simulink model "COMPLETO"  (R2024b)
settings: Solver=VariableStepAuto  StartTime=0.0  StopTime=10.0  RelTol=1e-3
undefined symbols (not defined in the file): ih, it, rhd, rtd
settings Model: Creator=ribei  LastModifiedBy=juani

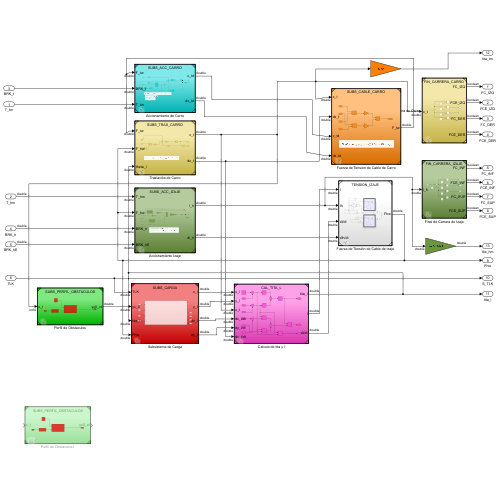
[thumbnail: Simulink's stored preview of the top-level diagram]
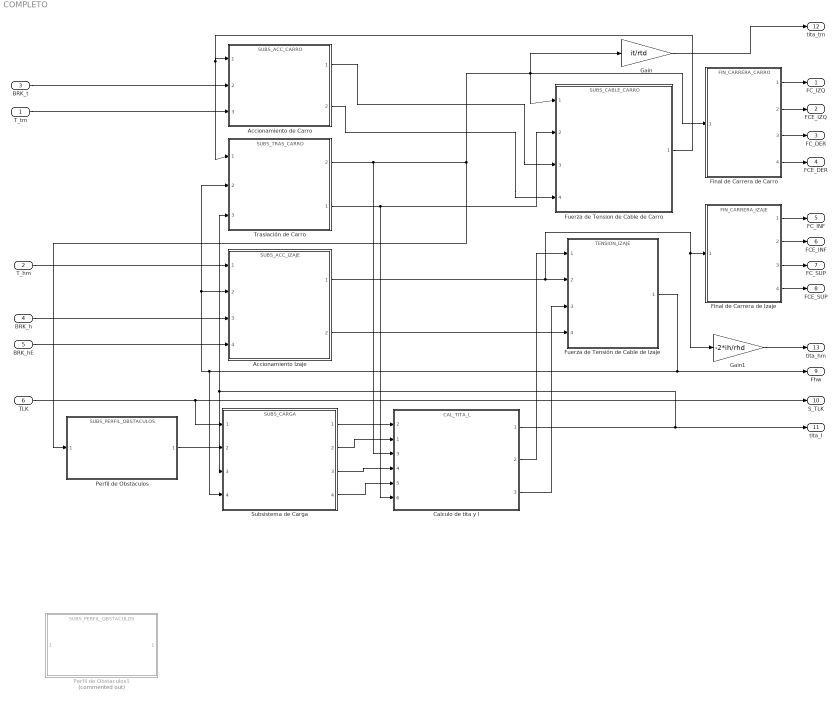
== system COMPLETO ==
  T_tm : Inport
  T_hm : Inport  Port=2
  BRK_t : Inport  Port=3
  BRK_h : Inport  Port=4
  BRK_hE : Inport  Port=5
  TLK : Inport  Port=6
  Accionamiento Izaje : ModelReference  ModelNameDialog=SUBS_ACC_IZAJE.slx  SimulationMode=Normal  ModelReferenceVersion=1.10
  Accionamiento de Carro : ModelReference  ModelNameDialog=SUBS_ACC_CARRO.slx  SimulationMode=Normal  ModelReferenceVersion=1.8
  Calculo de tita y l : ModelReference  ModelNameDialog=CAL_TITA_L.slx  SimulationMode=Normal  ModelReferenceVersion=4.0
      settings: PortSchema="{\"entries\":[{\"content\":{\"sides\":[{\"content\":{\"connectorIds\":[\"In2\",\"In1\",\"In3\",\"In4\",\"In5\",\"In6\"]},\"type\":\"ConnectorPlacement.EquallySpacedRectSide\",\"uuid\":\"8ead184c-a1e0-4b57-8217-57ade3346752\"},{\"content\":{\"connectorIds\":[\"Out1\",\"Out2\",\"Out3\"],\"side\":\"RIGHT\"},\"type\":\"ConnectorPlacement.EquallySpacedRectSide\",\"uuid\":\"562b51b5-55d8-4576-9d04-bf12fcd8d0f5\"},{\"content\":{\"side\":\"TOP\"},\"type\":\"ConnectorPlacement.EquallySpacedRectSide\",\"uuid\":\"2665fda4-9ae8-45ad-8675-5e3ba94dd8e3\"}]},\"type\":\"ConnectorPlacement.EquallySpacedConnector\",\"uuid\":\"240ee59b-efb7-462f-ad93-89fc511299ee\"}],\"packageUris\":[\"http://schema.mathworks.com/mf0/Connector/R2020b\"],\"version\":\"1.0\"}"
  Final de Carrera de Carro : ModelReference  ModelNameDialog=FIN_CARRERA_CARRO.slx  SimulationMode=Normal  ModelReferenceVersion=4.0
  Final de Carrera de Izaje : ModelReference  ModelNameDialog=FIN_CARRERA_IZAJE.slx  SimulationMode=Normal  ModelReferenceVersion=1.1
  Fuerza de Tension de Cable de Carro : ModelReference  ModelNameDialog=SUBS_CABLE_CARRO.slx  SimulationMode=Normal  ModelReferenceVersion=1.2
  Fuerza de Tensión de Cable de Izaje : ModelReference  ModelNameDialog=TENSION_IZAJE.slx  SimulationMode=Normal  ModelReferenceVersion=4.5
  Gain : Gain  Gain=it/rtd
  Gain1 : Gain  Gain=-2*ih/rhd
  Perfil de Obstaculos : ModelReference  ModelNameDialog=SUBS_PERFIL_OBSTACULOS.slx  SimulationMode=Normal  ModelReferenceVersion=1.76
  Perfil de Obstaculos1 : ModelReference  Commented=on  ModelNameDialog=SUBS_PERFIL_OBSTACULOS.slx  SimulationMode=Normal  ModelReferenceVersion=1.75
  Subsistema de Carga : ModelReference  ModelNameDialog=SUBS_CARGA.slx  SimulationMode=Normal  ModelReferenceVersion=1.25
  Traslación de Carro : ModelReference  ModelNameDialog=SUBS_TRAS_CARRO.slx  SimulationMode=Normal  ModelReferenceVersion=1.3
      settings: PortSchema="{\"entries\":[{\"content\":{\"sides\":[{\"content\":{\"connectorIds\":[\"In1\",\"In2\",\"In3\"]},\"type\":\"ConnectorPlacement.EquallySpacedRectSide\",\"uuid\":\"7b046cef-d788-43c7-aa6f-556876391631\"},{\"content\":{\"connectorIds\":[\"Out2\",\"Out1\"],\"side\":\"RIGHT\"},\"type\":\"ConnectorPlacement.EquallySpacedRectSide\",\"uuid\":\"be9a6f00-5e88-4651-bbf2-8ffe22406596\"},{\"content\":{\"side\":\"TOP\"},\"type\":\"ConnectorPlacement.EquallySpacedRectSide\",\"uuid\":\"81b3ad3c-f882-4752-9e65-d53dc15f63b3\"}]},\"type\":\"ConnectorPlacement.EquallySpacedConnector\",\"uuid\":\"5caf2ecc-c1ea-4fc8-a82b-392edb804ace\"}],\"packageUris\":[\"http://schema.mathworks.com/mf0/Connector/R2020b\"],\"version\":\"1.0\"}"
  FC_IZQ : Outport
  FCE_IZQ : Outport  Port=2
  FC_DER : Outport  Port=3
  FCE_DER : Outport  Port=4
  FC_INF : Outport  Port=5
  FCE_INF : Outport  Port=6
  FC_SUP : Outport  Port=7
  FCE_SUP : Outport  Port=8
  Fhw : Outport  Port=9
  S_TLK : Outport  Port=10
  tita_l : Outport  Port=11
  tita_tm : Outport  Port=12
  tita_hm : Outport  Port=13
  wires:
  Accionamiento Izaje/1 -> Fuerza de Tensión de Cable de Izaje/2, Gain1/1, Final de Carrera de Izaje/1
  Accionamiento Izaje/2 -> Fuerza de Tensión de Cable de Izaje/4
  Traslación de Carro/2 -> Calculo de tita y l/3, Perfil de Obstaculos/1, Gain/1, Final de Carrera de Carro/1, Fuerza de Tension de Cable de Carro/1
  Traslación de Carro/1 -> Calculo de tita y l/6, Fuerza de Tension de Cable de Carro/2
  Accionamiento de Carro/1 -> Fuerza de Tension de Cable de Carro/3
  Accionamiento de Carro/2 -> Fuerza de Tension de Cable de Carro/4
  T_tm/1 -> Accionamiento de Carro/3
  BRK_t/1 -> Accionamiento de Carro/2
  T_hm/1 -> Accionamiento Izaje/1
  BRK_h/1 -> Accionamiento Izaje/3
  BRK_hE/1 -> Accionamiento Izaje/4
  TLK/1 -> Subsistema de Carga/1, S_TLK/1
  Final de Carrera de Carro/1 -> FC_IZQ/1
  Final de Carrera de Carro/2 -> FCE_IZQ/1
  Final de Carrera de Carro/3 -> FC_DER/1
  Final de Carrera de Carro/4 -> FCE_DER/1
  Final de Carrera de Izaje/1 -> FC_INF/1
  Final de Carrera de Izaje/2 -> FCE_INF/1
  Final de Carrera de Izaje/3 -> FC_SUP/1
  Final de Carrera de Izaje/4 -> FCE_SUP/1
  Gain/1 -> tita_tm/1
  Gain1/1 -> tita_hm/1
  Perfil de Obstaculos/1 -> Subsistema de Carga/2
  Subsistema de Carga/1 -> Calculo de tita y l/2
  Subsistema de Carga/2 -> Calculo de tita y l/1
  Subsistema de Carga/3 -> Calculo de tita y l/4
  Subsistema de Carga/4 -> Calculo de tita y l/5
  Calculo de tita y l/1 -> Traslación de Carro/3, Subsistema de Carga/3, tita_l/1
  Fuerza de Tensión de Cable de Izaje/1 -> Accionamiento Izaje/2, Traslación de Carro/2, Subsistema de Carga/4, Fhw/1
  Calculo de tita y l/3 -> Fuerza de Tensión de Cable de Izaje/3
  Calculo de tita y l/2 -> Fuerza de Tensión de Cable de Izaje/1
  Fuerza de Tension de Cable de Carro/1 -> Traslación de Carro/1, Accionamiento de Carro/1
